simulink model "SingleTrackCANoe"  (R2021b)
settings: Solver=ode1  StartTime=0  StopTime=2  FixedStep=1.0000000000000000e-003  RelTol=1e-3
InitFcn:
  | sampleTime = str2double(get_param(bdroot, 'FixedStep'));
undefined symbols (not defined in the file or in its folder): AccPedalPos, BrakePedalPos, BrakeSwitch, DiscIntNeverNeededParam, DYNA4, EngSpd, IgnitionSwitch, InitialGear, InitialSpeed, IntendedEngTrq, LeftIndicator, MainBrakePress, MaxGear, MDL, MinGear, RefAcc, RefLane, RefLatPos, RefPath, RefPathCurv, RefSpd, RefSpdPreview, RefSpdRetrospect, RightIndicator, SteeringWheelAng, SteeringWheelTrq, UserDefinedRefValue, vm_const
libraries: UtilitiesLibrary x62, simulink x18, WheelSystemModules x14, LongitudinalControllerModules x13, LateralControllerModules x7, AnimationBusselectorModules x5, EnvironmentModules x5, BasicEngineControlModules x5, MiscellaneousControlModules x5, Animation3Modules x4, AuxiliariesModules x4, ReducedTireModules x4
(part 8 of 34)

== system SingleTrackCANoe/SimulationModel/VehicleControl/Miscellaneous ==
  note: How to add user-defined miscellaneous signals to the model:
      |
      | 1. Open the block "UserDefinedControlOutput" by double-clicking on it.
      | 2. Edit the signals inside by renaming them and setting the unit. You can also add signals to the existing ones.
      | 3. Adjust the size of the demux-block on the left of the bus-creator so that all ports can be connected.
      | 4. Save the model to apply your changes.
  Abscissae : Inport
  BrakeHydraulicsControl : MiscellaneousControlModules/BrakeHydraulicsControl  DATA_NODE=MDL.VehicleControl.Miscellaneous.BrakeHydraulicsControl  Circuit1PumpSignal=MDL.VehicleControl.Miscellaneous.BrakeHydraulicsControl.Circuit1PumpSignal  Circuit1PressReliefValveCurr=MDL.VehicleControl.Miscellaneous.BrakeHydraulicsControl.Circuit1PressReliefValveCurr  Circuit1ReversingValveCurr=MDL.VehicleControl.Miscellaneous.BrakeHydraulicsControl.Circuit1ReversingValveCurr  Circuit2PumpSignal=MDL.VehicleControl.Miscellaneous.BrakeHydraulicsControl.Circuit2PumpSignal  Circuit2PressReliefValveCurr=MDL.VehicleControl.Miscellaneous.BrakeHydraulicsControl.Circuit2PressReliefValveCurr  Circuit2ReversingValveCurr=MDL.VehicleControl.Miscellaneous.BrakeHydraulicsControl.Circuit2ReversingValveCurr  FrontLeftInletValveCurr=MDL.VehicleControl.Miscellaneous.BrakeHydraulicsControl.FrontLeftInletValveCurr  FrontLeftOutletValveCurr=MDL.VehicleControl.Miscellaneous.BrakeHydraulicsControl.FrontLeftOutletValveCurr  FrontRightInletValveCurr=MDL.VehicleControl.Miscellaneous.BrakeHydraulicsControl.FrontRightInletValveCurr  FrontRightOutletValveCurr=MDL.VehicleControl.Miscellaneous.BrakeHydraulicsControl.FrontRightOutletValveCurr  RearLeftInletValveCurr=MDL.VehicleControl.Miscellaneous.BrakeHydraulicsControl.RearLeftInletValveCurr  RearLeftOutletValveCurr=MDL.VehicleControl.Miscellaneous.BrakeHydraulicsControl.RearLeftOutletValveCurr  RearRightInletValveCurr=MDL.VehicleControl.Miscellaneous.BrakeHydraulicsControl.RearRightInletValveCurr  RearRightOutletValveCurr=MDL.VehicleControl.Miscellaneous.BrakeHydraulicsControl.RearRightOutletValveCurr
  Demux : Demux  Outputs=2
  DynaSystemInfo : Subsystem  Tag=DynaSystemInfo
      mask init:
      | data = get_param(gcb, 'UserData');
      settings: OpenFcn=DYNA4.ModelHandling.System.ShowEditSystemInformationDialog(gcb);
      mask Display: disp(['Type = ', data.type, '\nName = ', data.name ])
  EngineControl : MiscellaneousControlModules/EngineControl  DATA_NODE=MDL.VehicleControl.Miscellaneous.EngineControl  RefEngSpd=MDL.VehicleControl.Miscellaneous.EngineControl.RefEngSpd  EngTrq=MDL.VehicleControl.Miscellaneous.EngineControl.EngTrq  FuelMass=MDL.VehicleControl.Miscellaneous.EngineControl.FuelMass  AftercoolerOutAirTemp=MDL.VehicleControl.Miscellaneous.EngineControl.AftercoolerOutAirTemp  IgnitionAng=MDL.VehicleControl.Miscellaneous.EngineControl.IgnitionAng  ThrottlePos=MDL.VehicleControl.Miscellaneous.EngineControl.ThrottlePos  ThrottleMassFlow=MDL.VehicleControl.Miscellaneous.EngineControl.ThrottleMassFlow  InjectionMassPre=MDL.VehicleControl.Miscellaneous.EngineControl.InjectionMassPre  InjectionMassMain=MDL.VehicleControl.Miscellaneous.EngineControl.InjectionMassMain  InjectionMassPost1=MDL.VehicleControl.Miscellaneous.EngineControl.InjectionMassPost1  InjectionMassPost2=MDL.VehicleControl.Miscellaneous.EngineControl.InjectionMassPost2  InjectionAngPre=MDL.VehicleControl.Miscellaneous.EngineControl.InjectionAngPre  InjectionAngMain=MDL.VehicleControl.Miscellaneous.EngineControl.InjectionAngMain  InjectionAngPost1=MDL.VehicleControl.Miscellaneous.EngineControl.InjectionAngPost1  InjectionAngPost2=MDL.VehicleControl.Miscellaneous.EngineControl.InjectionAngPost2  IntakeCamOffsetAng=MDL.VehicleControl.Miscellaneous.EngineControl.IntakeCamOffsetAng  ExhaustCamOffsetAng=MDL.VehicleControl.Miscellaneous.EngineControl.ExhaustCamOffsetAng  RelativeOpeningEGRValve=MDL.VehicleControl.Miscellaneous.EngineControl.RelativeOpeningEGRValve  Load=MDL.VehicleControl.Miscellaneous.EngineControl.Load
  SuspensionTestRigControl : MiscellaneousControlModules/SuspensionTestRigControl  DATA_NODE=MDL.VehicleControl.Miscellaneous.SuspensionTestRigControl  ClampSwitch=MDL.VehicleControl.Miscellaneous.SuspensionTestRigControl.ClampSwitch
  TemperatureControl : MiscellaneousControlModules/TemperatureControl  DATA_NODE=MDL.VehicleControl.Miscellaneous.TemperatureControl  TransmissionTemp=MDL.VehicleControl.Miscellaneous.TemperatureControl.TransmissionTemp  GearStageTemp=MDL.VehicleControl.Miscellaneous.TemperatureControl.GearStageTemp  TransferCaseTemp=MDL.VehicleControl.Miscellaneous.TemperatureControl.TransferCaseTemp  FrontDifferentialTemp=MDL.VehicleControl.Miscellaneous.TemperatureControl.FrontDifferentialTemp  RearDifferentialTemp=MDL.VehicleControl.Miscellaneous.TemperatureControl.RearDifferentialTemp  RearTransferCaseTemp=MDL.VehicleControl.Miscellaneous.TemperatureControl.RearTransferCaseTemp  Rear2DifferentialTemp=MDL.VehicleControl.Miscellaneous.TemperatureControl.Rear2DifferentialTemp  Rear3DifferentialTemp=MDL.VehicleControl.Miscellaneous.TemperatureControl.Rear3DifferentialTemp  ElecMotorTemp=MDL.VehicleControl.Miscellaneous.TemperatureControl.ElecMotorTemp  GeneratorTemp=MDL.VehicleControl.Miscellaneous.TemperatureControl.GeneratorTemp  CoolantTemp=MDL.VehicleControl.Miscellaneous.TemperatureControl.CoolantTemp
  UserDefinedControl : MiscellaneousControlModules/UserDefinedControl  DATA_NODE=MDL.VehicleControl.Miscellaneous.UserDefinedControl
  UserDefinedControlOutput : Subsystem  Tag=TESIS DYNAware Interface Block  mask{NeedsUpdate=off, SignalInfo=|}
      mask SignalInfo=|
      | {
      |   "Version": "4.6",
      |   "MuxedOutputBusName": "UserDefinedControl",
      |   "MuxedInputBusName": "fromCTRL",
      |   "MuxedInputSelected": false,
      |   "MuxedOutputSelected": true,
      |   "SignalData": [
      |     {
      |       "initialValue": "0.0",
      |       "name": "UserDefined1[-]",
      |       "comment": "User-defined miscellaneous signal 1 (can be edited by the user) ",
      |       "minString": "",
      |       "maxString": "",
      |       "width": 1,
      |       "dataType": 0,
      |       "signalType": 0,
      |       "createSignal": false,
      |       "outputName": "UserDefined1[-]",
      |       "generateSignalAccessBlock": false,
      |       "accessId": "$(parentId).$(blockName).$(outputName)"
      |     },
      |     {
      |       "initialValue": "0.0",
      |       "name": "UserDefined2[-]",
      |       "comment": "User-defined miscellaneous signal 2 (can be edited by the user) ",
      |       "minString": "",
      |       "maxString": "",
      |       "width": 1,
      |       "dataType": 0,
      |       "signalType": 0,
      |       "createSignal": false,
      |       "outputName": "UserDefined2[-]",
      |       "generateSignalAccessBlock": false,
      |       "accessId": "$(parentId).$(blockName).$(outputName)"
      |     }
      |   ]
      | }
      mask prompts: NeedsUpdate "Specify, if subsystem content needs to be updated"; SignalInfo "Signal Info (json)"
      mask help: DYNA4 Interface Block Version 4.6
      mask init:
      | blockName = get_param(gcbh, 'Name');
      | parentId = DYNA4.ModelHandling.AccessID.getFromHierarchy(gcbh);
      | TD.InterfaceBlock.ModelCallbacks.GenerateContent(gcb);
      settings: DeleteFcn=TD.InterfaceBlock.ModelCallbacks.CloseGUI( gcbh );  NameChangeFcn=TD.InterfaceBlock.ModelCallbacks.BlockRenamedHandler(gcbh);  OpenFcn=TD.InterfaceBlock.ModelCallbacks.OpenGUI( gcbh );  CloseFcn=TD.InterfaceBlock.ModelCallbacks.CloseGUI( gcbh );
      mask Display:
      | image('InterfaceBlock.png','center');
      | port_label('input',1, 'UserDefined1[-]');
      | port_label('input',2, 'UserDefined2[-]');
      | port_label('output',1, 'UserDefinedControl');
  BrakeHydraulicsParams : Outport  VectorParamsAs1DForOutWhenUnconnected=off
  EngineControlParams : Outport  Port=2  VectorParamsAs1DForOutWhenUnconnected=off
  SuspensionTestRigControlParams : Outport  Port=3  VectorParamsAs1DForOutWhenUnconnected=off
  TemperatureControlParams : Outport  Port=4  VectorParamsAs1DForOutWhenUnconnected=off
  UserDefinedControlParams : Outport  Port=5  VectorParamsAs1DForOutWhenUnconnected=off
  wires:
  Demux/2 -> UserDefinedControlOutput/2(UserDefined2[-]___UNIQUE_1)
  Demux/1 -> UserDefinedControlOutput/1(UserDefined1[-]___UNIQUE_1)
  UserDefinedControl/1 -> Demux/1
  UserDefinedControlOutput/1(UserDefinedControl___UNIQUE_1) -> UserDefinedControlParams/1
  Abscissae/1 -> EngineControl/1, UserDefinedControl/1, TemperatureControl/1, SuspensionTestRigControl/1, BrakeHydraulicsControl/1
  BrakeHydraulicsControl/1 -> BrakeHydraulicsParams/1
  EngineControl/1 -> EngineControlParams/1
  SuspensionTestRigControl/1 -> SuspensionTestRigControlParams/1
  TemperatureControl/1 -> TemperatureControlParams/1
